simulink model "FIXEDPOINT_SECOND_ORDER_SIGMADELTA"  (R2021b)
settings: Solver=VariableStepAuto  StartTime=0.0  StopTime=0.01  MaxStep=1e-8  RelTol=1e-3
libraries: fl_lib x9, nesl_utility x4
settings Model: Creator=caccolillo  LastModifiedBy=caccolillo
settings OptimizationCC: BlockReduction=off  ConditionallyExecuteInputs=off
settings DebuggingCC: SignalRangeChecking=warning

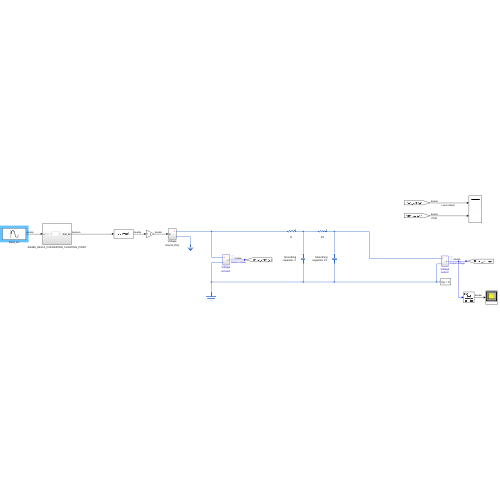
[thumbnail: Simulink's stored preview of the top-level diagram]
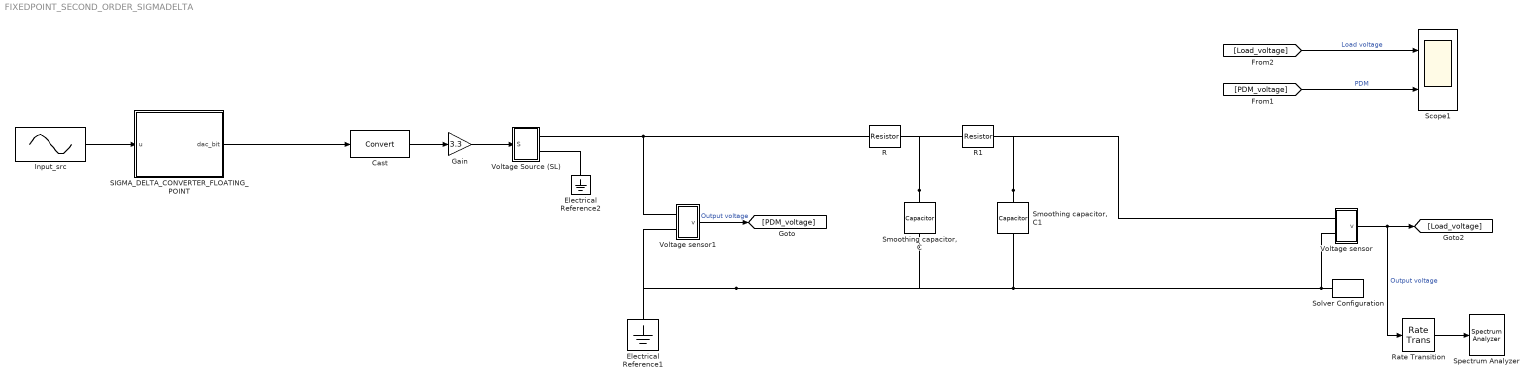
== system FIXEDPOINT_SECOND_ORDER_SIGMADELTA ==
  Cast : DataTypeConversion
  Electrical Reference1 : fl_lib/Electrical/Electrical Elements/Electrical Reference
  Electrical Reference2 : fl_lib/Electrical/Electrical Elements/Electrical Reference
  Gain : Gain  Gain=3.3
  Input_src : Sin  Amplitude=1024  Frequency=2*pi*1000  SampleTime=2e-07
  R : fl_lib/Electrical/Electrical Elements/Resistor  R=1 kOhm  i_specify=off  i_priority=High  i=0 A  i_nominal_specify=off  i_nominal_unit=A  i_nominal_value=1  v_specify=off  v_priority=High  v=0 V  v_nominal_specify=off  v_nominal_unit=V  v_nominal_value=1
  R1 : fl_lib/Electrical/Electrical Elements/Resistor  R=1 kOhm  i_specify=off  i_priority=High  i=0 A  i_nominal_specify=off  i_nominal_unit=A  i_nominal_value=1  v_specify=off  v_priority=High  v=0 V  v_nominal_specify=off  v_nominal_unit=V  v_nominal_value=1
  Rate Transition : RateTransition  Deterministic=off  OutPortSampleTime=1/100e3
  SIGMA_DELTA_CONVERTER_FLOATING_POINT : Subsystem
  Scope1 : Scope  NumInputPorts=2
  "Smoothing capacitor, C" : fl_lib/Electrical/Electrical Elements/Capacitor  c=10 nF  r=0 Ohm  g=0 1/Ohm  i_specify=off  i_priority=High  i=0 A  i_nominal_specify=off  i_nominal_unit=A  i_nominal_value=1  v_specify=off  v_priority=High  v=0 V  v_nominal_specify=off  v_nominal_unit=V  v_nominal_value=1  vc_specify=on  vc_priority=High  vc=0 V  vc_nominal_specify=off  vc_nominal_unit=V  vc_nominal_value=1
  "Smoothing capacitor, C1" : fl_lib/Electrical/Electrical Elements/Capacitor  c=10 nF  r=0 Ohm  g=0 1/Ohm  i_specify=off  i_priority=High  i=0 A  i_nominal_specify=off  i_nominal_unit=A  i_nominal_value=1  v_specify=off  v_priority=High  v=0 V  v_nominal_specify=off  v_nominal_unit=V  v_nominal_value=1  vc_specify=on  vc_priority=High  vc=0 V  vc_nominal_specify=off  vc_nominal_unit=V  vc_nominal_value=1
  Solver Configuration : nesl_utility/Solver Configuration  PhysicalDomain=network_engine_domain  SubClassName=solver  LeftPortType=input  RightPortType=generic  Tones=[]  Harmonics=[]  SimulateNoise=off  Profile=off  UseLocalSampling=off  EnableSwitchedLinearOptims=on  FrequencyDomain=off  UseCCode=off  RelTol=0.001  AbsTol=1e-06  MinStep=1e-09  ToWorkspace=off  RevertToSquareIcSolve=off  NumHomotopyIterations=100  PhasorMode=off  PhasorModeNumHarmonics=1  DoDC=off  ResidualTolerance=1e-9  UseLocalSolver=off  LocalSolverChoice=NE_BACKWARD_EULER_ADVANCER  LocalSolverSampleTime=1e-7  DoFixedCost=off  MaxNonlinIter=12  MaxModeIter=2  ComputeImpulses=off  ImpulseIterations=2  LinearAlgebra=Sparse  EquationFormulation=NE_TIME_EF  DelaysMemoryBudget=1024  AutomaticFiltering=on  FilteringTimeConstant=0.001  PartitionStorageMethod=AS_NEEDED  PartitionMemoryBudget=1024  PartitionMethod=FAST
      settings: SourceProductBaseCode=PW,SS
  Spectrum Analyzer : SpectrumAnalyzer
  Voltage Source (SL) : Subsystem
      settings: CopyFcn=set_param(gcb,'LinkStatus','none')
  Voltage sensor : Subsystem
      settings: CopyFcn=set_param(gcb,'LinkStatus','none')
  Voltage sensor1 : Subsystem
      settings: CopyFcn=set_param(gcb,'LinkStatus','none')
  wires:
  [PDM_voltage] -> Scope1/2  "PDM"
  Rate Transition/1 -> Spectrum Analyzer/1
  Voltage sensor/1(v) -> Rate Transition/1, [Load_voltage]  "Output voltage"
  Voltage sensor1/1(v) -> [PDM_voltage]  "Output voltage"
  Gain/1 -> Voltage Source (SL)/1(S)
  [Load_voltage] -> Scope1/1  "Load voltage"
  Cast/1 -> Gain/1
  Input_src/1 -> SIGMA_DELTA_CONVERTER_FLOATING_POINT/1(u)
  SIGMA_DELTA_CONVERTER_FLOATING_POINT/1(dac_bit) -> Cast/1
  connections:
  Solver Configuration/RConn1 -- Voltage sensor1/LConn2 -- Electrical Reference1/LConn1 -- "Smoothing capacitor, C"/RConn1 -- "Smoothing capacitor, C1"/RConn1 -- Voltage sensor/LConn2
  "Smoothing capacitor, C"/LConn1 -- R/LConn1 -- R1/RConn1
  "Smoothing capacitor, C1"/LConn1 -- R1/LConn1 -- Voltage sensor/LConn1
  Voltage sensor1/LConn1 -- R/RConn1 -- Voltage Source (SL)/RConn1
  Voltage Source (SL)/RConn2 -- Electrical Reference2/LConn1

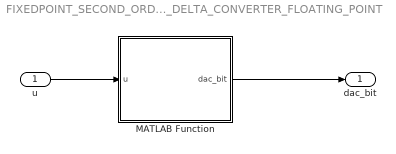
== system FIXEDPOINT_SECOND_ORDER_SIGMADELTA/SIGMA_DELTA_CONVERTER_FLOATING_POINT ==
  u : Inport
  MATLAB Function : MATLAB Function  TreatAsAtomicUnit=on
  dac_bit : Outport
  wires:
  u/1 -> MATLAB Function/1(u)
  MATLAB Function/1(dac_bit) -> dac_bit/1

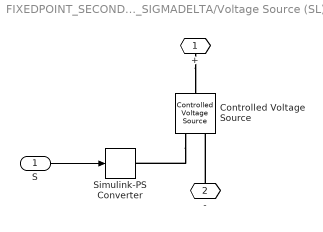
== system FIXEDPOINT_SECOND_ORDER_SIGMADELTA/Voltage Source (SL) ==
  S : Inport
  Controlled Voltage Source : fl_lib/Electrical/Electrical Sources/Controlled Voltage Source
  Simulink-PS Converter : nesl_utility/Simulink-PS Converter  PhysicalDomain=network_engine_domain  SubClassName=ps_input  LeftPortType=input  RightPortType=output  PseudoPeriodic=off  Frequencies=[]  NoiseDistribution=none  NoiseParameters=[]  Unit=V  AffineConversion=off  FilteringAndDerivatives=zero  SimscapeFilterOrder=1  InputFilterTimeConstant=.001  UdotUserProvided=0
      settings: SourceProductBaseCode=PW,SS
  + : PMIOPort  Side=Right
  - : PMIOPort  Port=2  Side=Right
  wires:
  S/1 -> Simulink-PS Converter/1
  connections:
  +/RConn1 -- Controlled Voltage Source/LConn1
  -/RConn1 -- Controlled Voltage Source/RConn2
  Controlled Voltage Source/RConn1 -- Simulink-PS Converter/RConn1

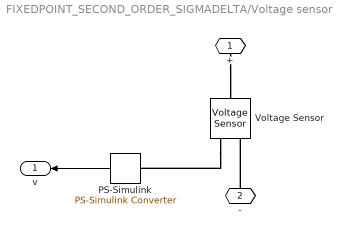
== system FIXEDPOINT_SECOND_ORDER_SIGMADELTA/Voltage sensor ==
  PS-Simulink : nesl_utility/PS-Simulink Converter  PhysicalDomain=network_engine_domain  SubClassName=ps_output  LeftPortType=input  RightPortType=output  PseudoPeriodic=off  Frequencies=[]  Unit=V  AffineConversion=off
      settings: SourceProductBaseCode=PW,SS
  Voltage Sensor : fl_lib/Electrical/Electrical Sensors/Voltage Sensor
  + : PMIOPort  Side=Left
  - : PMIOPort  Port=2  Side=Left
  v : Outport
  wires:
  PS-Simulink/1 -> v/1
  connections:
  Voltage Sensor/RConn1 -- PS-Simulink/LConn1
  +/RConn1 -- Voltage Sensor/LConn1
  -/RConn1 -- Voltage Sensor/RConn2

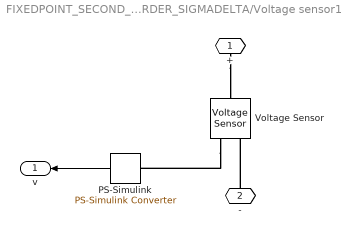
== system FIXEDPOINT_SECOND_ORDER_SIGMADELTA/Voltage sensor1 ==
  PS-Simulink : nesl_utility/PS-Simulink Converter  PhysicalDomain=network_engine_domain  SubClassName=ps_output  LeftPortType=input  RightPortType=output  PseudoPeriodic=off  Frequencies=[]  Unit=V  AffineConversion=off
      settings: SourceProductBaseCode=PW,SS
  Voltage Sensor : fl_lib/Electrical/Electrical Sensors/Voltage Sensor
  + : PMIOPort  Side=Left
  - : PMIOPort  Port=2  Side=Left
  v : Outport
  wires:
  PS-Simulink/1 -> v/1
  connections:
  Voltage Sensor/RConn1 -- PS-Simulink/LConn1
  +/RConn1 -- Voltage Sensor/LConn1
  -/RConn1 -- Voltage Sensor/RConn2

== matlab function FIXEDPOINT_SECOND_ORDER_SIGMADELTA/SIGMA_DELTA_CONVERTER_FLOATING_POINT/MATLAB Function ==
  data: u input; dac_bit output
function dac_bit = SDM_fcn_fp(u)  %#codegen

%% 2nd-order CIFB SDM — double-precision floating-point version
%% u is the audio sample input — same scale as the integer version:
%%   range -4096 to +4095 (13-bit signed full scale)
%%
%% All internal arithmetic uses double precision.
%% Coefficients are the same Q16 integer values divided by 2^16
%% so they represent the same real-valued coefficients as the
%% Verilog/integer implementation.
%%
%% Output: boolean dac_bit (1-bit PDM)

dac_bit = false;

persistent int1 int2
if isempty(int1)
    int1 = 0.0;
    int2 = 0.0;
end

%% ---------------------------------------------------------------
%  COEFFICIENTS — exact same values as integer version
%  Original integers were Q16 (scaled by 2^16 = 65536)
%  Dividing by 65536 recovers the real-valued coefficient
% ---------------------------------------------------------------
B1 = 51138 / 65536;     %  ≈ 0.7803
A1 = 51138 / 65536;     %  ≈ 0.7803
C1 =  3493 / 65536;     %  ≈ 0.0533
A2 =  9765 / 65536;     %  ≈ 0.1490

%% ---------------------------------------------------------------
%  INPUT NORMALISATION
%  Map the 13-bit signed integer input to the [-1, +1] range
%  expected by the normalised SDM coefficients above.
%
%  +4095 → +0.9998
%  -4096 → -1.0
% ---------------------------------------------------------------
u_d = double(u);

%% Clamp to 13-bit signed range
if u_d >  4095, u_d =  4095; end
if u_d < -4096, u_d = -4096; end

%% Normalise to [-1, +1]
u_norm = u_d / 4096.0;

%% ---------------------------------------------------------------
%  QUANTIZER — sign of int2
% ---------------------------------------------------------------
if int2 >= 0.0
    dac_bit = true;
    dac_val = +1.0;
else
    dac_bit = false;
    dac_val = -1.0;
end

%% ---------------------------------------------------------------
%  INTEGRATOR 1: int1[n] = B1*u_norm[n] + int1[n-1] - A1*dac_val
% ---------------------------------------------------------------
int1 = int1 + B1 * u_norm - A1 * dac_val;

%% Saturation — match integer version's ±524288/65536 = ±8.0 range
if int1 >  8.0, int1 =  8.0; end
if int1 < -8.0, int1 = -8.0; end

%% ---------------------------------------------------------------
%  INTEGRATOR 2: int2[n] = C1*int1[n] + int2[n-1] - A2*dac_val
% ---------------------------------------------------------------
int2 = int2 + C1 * int1 - A2 * dac_val;

%% Saturation
if int2 >  8.0, int2 =  8.0; end
if int2 < -8.0, int2 = -8.0; end

end
